simulink model "LMOpenLoop(1)"  (R2014a)
settings: Solver=ode45  StartTime=0.0  StopTime=4  MaxStep=0.0034  RelTol=1e-6
libraries: simulink x2
settings Model: Creator=Daniel  LastModifiedBy=Daniel
settings SolverCC: ConsecutiveZCsStepRelTol=10*64*eps
settings DataIOCC: LimitDataPoints=off  Refine=20

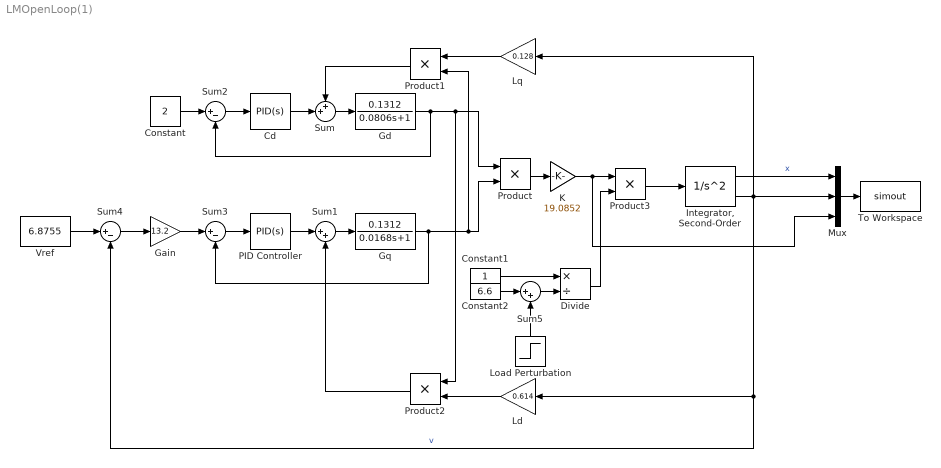
== system LMOpenLoop(1) ==
  Cd : simulink/Continuous/PID Controller  Controller=PID  TimeDomain=Continuous-time  SampleTime=1  IntegratorMethod=Forward Euler  FilterMethod=Forward Euler  Form=Parallel  P=18.7  I=279  D=0.05  N=100  InitialConditionSource=internal  InitialConditionForIntegrator=0  InitialConditionForFilter=0  ExternalReset=none  LimitOutput=off  UpperSaturationLimit=inf  LowerSaturationLimit=-inf  LinearizeAsGain=on  AntiWindupMode=none  Kb=1  TrackingMode=off  Kt=1  PParamMin=[]  PParamMax=[]  IParamMin=[]  IParamMax=[]  DParamMin=[]  DParamMax=[]  NParamMin=[]  NParamMax=[]  KbParamMin=[]  KbParamMax=[]  KtParamMin=[]  KtParamMax=[]  POutMin=[]  POutMax=[]  IOutMin=[]  IOutMax=[]  DOutMin=[]  DOutMax=[]  NOutMin=[]  NOutMax=[]  KbOutMin=[]  KbOutMax=[]  KtOutMin=[]  KtOutMax=[]  IntegratorOutMin=[]  IntegratorOutMax=[]  FilterOutMin=[]  FilterOutMax=[]  SumOutMin=[]  SumOutMax=[]  SumI1OutMin=[]  SumI1OutMax=[]  SumI2OutMin=[]  SumI2OutMax=[]  SumI3OutMin=[]  SumI3OutMax=[]  SumDOutMin=[]  SumDOutMax=[]  SaturationOutMin=[]  SaturationOutMax=[]  IntegratorContinuousStateAttributes=''  IntegratorStateMustResolveToSignalObject=off  IntegratorRTWStateStorageClass=Auto  FilterContinuousStateAttributes=''  FilterStateMustResolveToSignalObject=off  FilterRTWStateStorageClass=Auto
  Constant : Constant  Value=2
  Constant1 : Constant
  Constant2 : Constant  Value=6.6
  Divide : Product  Inputs=*/
  Gain : Gain  Gain=13.2
  Gd : TransferFcn  Numerator=[0.1312]  Denominator=[0.0806 1]
  Gq : TransferFcn  Numerator=[0.1312]  Denominator=[0.0168 1]
  "Integrator, Second-Order" : SecondOrderIntegrator  ICDXDT=6.8755
  K : Gain  Gain=19.0852
  Ld : Gain  Gain=0.614
  Load Perturbation : Step  Time=2  After=10  SampleTime=0
  Lq : Gain  Gain=0.128
  Mux : Mux  Inputs=3
  PID Controller : simulink/Continuous/PID Controller  Controller=PID  TimeDomain=Continuous-time  SampleTime=1  IntegratorMethod=Forward Euler  FilterMethod=Forward Euler  Form=Parallel  P=4.5  I=289  D=0.017  N=100  InitialConditionSource=internal  InitialConditionForIntegrator=0  InitialConditionForFilter=0  ExternalReset=none  LimitOutput=off  UpperSaturationLimit=inf  LowerSaturationLimit=-inf  LinearizeAsGain=on  AntiWindupMode=none  Kb=1  TrackingMode=off  Kt=1  PParamMin=[]  PParamMax=[]  IParamMin=[]  IParamMax=[]  DParamMin=[]  DParamMax=[]  NParamMin=[]  NParamMax=[]  KbParamMin=[]  KbParamMax=[]  KtParamMin=[]  KtParamMax=[]  POutMin=[]  POutMax=[]  IOutMin=[]  IOutMax=[]  DOutMin=[]  DOutMax=[]  NOutMin=[]  NOutMax=[]  KbOutMin=[]  KbOutMax=[]  KtOutMin=[]  KtOutMax=[]  IntegratorOutMin=[]  IntegratorOutMax=[]  FilterOutMin=[]  FilterOutMax=[]  SumOutMin=[]  SumOutMax=[]  SumI1OutMin=[]  SumI1OutMax=[]  SumI2OutMin=[]  SumI2OutMax=[]  SumI3OutMin=[]  SumI3OutMax=[]  SumDOutMin=[]  SumDOutMax=[]  SaturationOutMin=[]  SaturationOutMax=[]  IntegratorContinuousStateAttributes=''  IntegratorStateMustResolveToSignalObject=off  IntegratorRTWStateStorageClass=Auto  FilterContinuousStateAttributes=''  FilterStateMustResolveToSignalObject=off  FilterRTWStateStorageClass=Auto
  Product{,1..3} (4 alike) : Product
  Sum : Sum  Inputs=++|
  Sum1 : Sum  Inputs=|++
  Sum2 : Sum  Inputs=|+-
  Sum3 : Sum  Inputs=|+-
  Sum4 : Sum  Inputs=|+-
  Sum5 : Sum  Inputs=|++
  To Workspace : ToWorkspace  VariableName=simout  SaveFormat=Timeseries  SampleTime=-1
  Vref : Constant  Value=6.8755
  wires:
  Gd/1 -> Sum2/2, Product2/1, Product/1
  Gq/1 -> Sum3/2, Product1/2, Product/2
  Product/1 -> K/1
  "Integrator, Second-Order"/1 -> Mux/1  "x"
  "Integrator, Second-Order"/2 -> Lq/1, Mux/2, Ld/1, Sum4/2  "v"
  Lq/1 -> Product1/1
  Product1/1 -> Sum/1
  Sum/1 -> Gd/1
  Ld/1 -> Product2/2
  Product2/1 -> Sum1/2
  Sum1/1 -> Gq/1
  Mux/1 -> To Workspace/1
  PID Controller/1 -> Sum1/1
  Cd/1 -> Sum/2
  Sum2/1 -> Cd/1
  Constant/1 -> Sum2/1
  Sum3/1 -> PID Controller/1
  Gain/1 -> Sum3/1
  Sum4/1 -> Gain/1
  Vref/1 -> Sum4/1
  Product3/1 -> "Integrator, Second-Order"/1
  K/1 -> Mux/3, Product3/1
  Constant1/1 -> Divide/1
  Sum5/1 -> Divide/2
  Divide/1 -> Product3/2
  Constant2/1 -> Sum5/1
  Load Perturbation/1 -> Sum5/2
